simulink model "MCP_phase2_nonlinear_simulink"  (R2020a)
settings: Solver=VariableStepAuto  StartTime=0.0  StopTime=1000  RelTol=1e-3
values from neighbouring files (symbols this model uses):
  eq_values = zeros(4,1)    [MCP_phase2_nonlinear.m]
  h1_eq = 11.4    [MCP_phase2_linear.m]    (also in MCP_phase2_nonlinear.m)
  h2_eq = 11.6    [MCP_phase2_linear.m]    (also in MCP_phase2_nonlinear.m)
  h3_eq = 5.3    [MCP_phase2_linear.m]    (also in MCP_phase2_nonlinear.m)
  h4_eq = 4    [MCP_phase2_linear.m]    (also in MCP_phase2_nonlinear.m)
settings Model: Creator=rafiee  LastModifiedBy=Lenovo
settings DataIOCC: ReturnWorkspaceOutputs=off
settings DebuggingCC: ArithmeticOperatorsInVariantConditions=warning
settings SFSimCC: SimUseLocalCustomCode=off  CustomCodeUndefinedFunction=UseInterfaceOnly
settings RTWCC: RTWUseLocalCustomCode=off
settings CodeAppCC: StateflowObjectComments=on

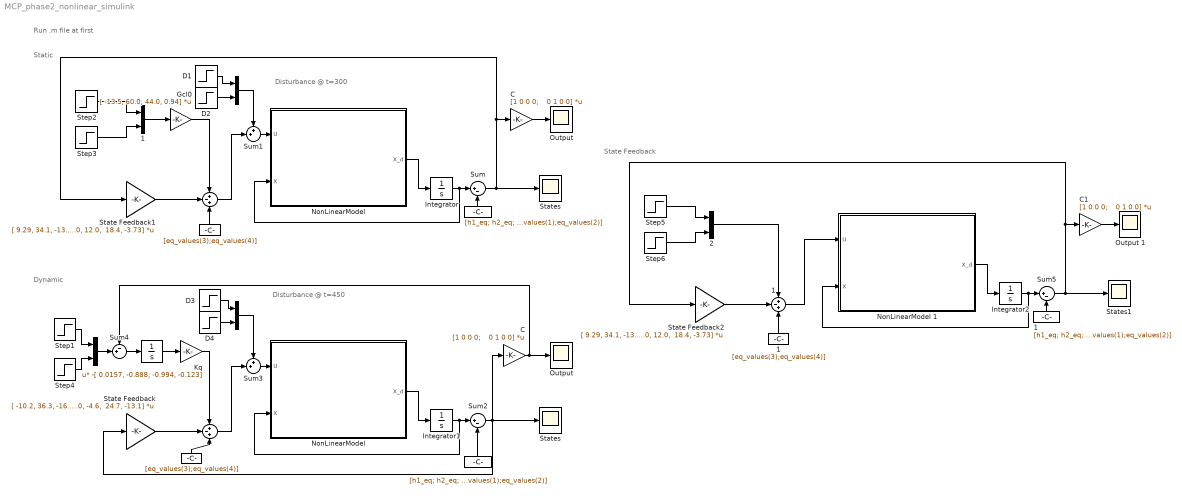
== system MCP_phase2_nonlinear_simulink ==
  note: State Feedback
  note: Run .m file at first
  note: Static
  note: Dynamic
  note: Disturbance @ t=450
  note: Disturbance @ t=300
  " " : Integrator
  " " : Sum  Inputs=+-+
  "      " : Concatenate
  "        " : Sum  Inputs=+-+
  "                        " : Constant  Value=[eq_values(3);eq_values(4)]
  "                             " : Constant  Value=[h1_eq; h2_eq; eq_values(1);eq_values(2)]
  " " : Constant  Value=[h1_eq; h2_eq; eq_values(1);eq_values(2)]
  "                                  " : Constant  Value=[eq_values(3);eq_values(4)]
  "                                                                   " : Concatenate
  "                                                                         " : Concatenate
  "                             1" : Constant  Value=[h1_eq; h2_eq; eq_values(1);eq_values(2)]
  "                        1" : Constant  Value=[eq_values(3);eq_values(4)]
  "        1" : Sum  Inputs=+-+
  "   1" : Concatenate
  "   2" : Concatenate
  C : Gain  Gain=|  Multiplication=Matrix(K*u)
      | [1 0 0 0;
      |    0 1 0 0]
  "C  " : Gain  Gain=|  Multiplication=Matrix(K*u)
      | [1 0 0 0;
      |    0 1 0 0]
  C1 : Gain  Gain=|  Multiplication=Matrix(K*u)
      | [1 0 0 0;
      |    0 1 0 0]
  D1 : Step  Time=300  After=4  SampleTime=0
  D2 : Step  Time=300  After=4  SampleTime=0
  D3 : Step  Time=450  After=4  SampleTime=0
  D4 : Step  Time=450  After=4  SampleTime=0
  Gcl0 : Gain  Gain=[ -13.5, 60.0; 44.0, 0.94]  Multiplication=Matrix(K*u)
  Integrator : Integrator  InitialCondition=[h1_eq;h2_eq;h3_eq;h4_eq]
  Integrator1 : Integrator  InitialCondition=[h1_eq;h2_eq;h3_eq;h4_eq]
  Integrator2 : Integrator  InitialCondition=[h1_eq;h2_eq;h3_eq;h4_eq]
  Kq : Gain  Gain=-[ 0.0157, -0.888; -0.994, -0.123]  Multiplication=Matrix(u*K)
  NonLinearModel : MATLAB Function  TreatAsAtomicUnit=on
  "NonLinearModel " : MATLAB Function  TreatAsAtomicUnit=on
  NonLinearModel 1 : MATLAB Function  TreatAsAtomicUnit=on
  "Output " : Scope
  Output 1 : Scope
  "Output  " : Scope
  "State Feedback " : Gain  Gain="[ -10.2, 36.3, -16.5,  24.5; 41.0, -4.6,  24.7, -13.1]"  Multiplication=Matrix(K*u)
  State Feedback1 : Gain  Gain="[ 9.29, 34.1, -13.6,  24.9; 23.0, 12.0,  18.4, -3.73]"  Multiplication=Matrix(K*u)
  State Feedback2 : Gain  Gain="[ 9.29, 34.1, -13.6,  24.9; 23.0, 12.0,  18.4, -3.73]"  Multiplication=Matrix(K*u)
  States : Scope
  "States " : Scope
  States1 : Scope
  Step{1..6} (6 alike) : Step  SampleTime=0
  Sum : Sum  Inputs=|+-
  Sum1 : Sum  Inputs=++|
  Sum2 : Sum  Inputs=|+-
  Sum3 : Sum  Inputs=++|
  Sum4 : Sum  Inputs=-+|
  Sum5 : Sum  Inputs=|+-
  wires:
  "                             "/1 -> Sum/2
  Integrator/1 -> Sum/1, "NonLinearModel "/2(X)
  Gcl0/1 -> "        "/1
  "NonLinearModel "/1(X_d) -> Integrator/1
  "   1"/1 -> Gcl0/1
  State Feedback1/1 -> "        "/2
  "                        "/1 -> "        "/3
  Step3/1 -> "   1"/2
  Step2/1 -> "   1"/1
  C/1 -> "Output "/1
  Sum/1 -> C/1, State Feedback1/1, States/1
  D1/1 -> "                                                                   "/1
  D2/1 -> "                                                                   "/2
  "                                                                   "/1 -> Sum1/1
  Sum1/1 -> "NonLinearModel "/1(U)
  "        "/1 -> Sum1/2
  "C  "/1 -> "Output  "/1, Sum4/1
  "      "/1 -> Sum4/2
  Sum4/1 -> " "/1
  Sum2/1 -> "State Feedback "/1, "States "/1, "C  "/1
  Step1/1 -> "      "/1
  Step4/1 -> "      "/2
  D3/1 -> "                                                                         "/1
  D4/1 -> "                                                                         "/2
  "State Feedback "/1 -> " "/2
  "                                                                         "/1 -> Sum3/1
  " "/1 -> Sum3/2
  NonLinearModel/1(X_d) -> Integrator1/1
  Kq/1 -> " "/1
  " "/1 -> Sum2/2
  " "/1 -> Kq/1
  Integrator1/1 -> Sum2/1, NonLinearModel/2(X)
  Sum3/1 -> NonLinearModel/1(U)
  "                                  "/1 -> " "/3
  Step6/1 -> "   2"/2
  Step5/1 -> "   2"/1
  C1/1 -> Output 1/1
  State Feedback2/1 -> "        1"/2
  Sum5/1 -> C1/1, State Feedback2/1, States1/1
  NonLinearModel 1/1(X_d) -> Integrator2/1
  Integrator2/1 -> Sum5/1, NonLinearModel 1/2(X)
  "                             1"/1 -> Sum5/2
  "                        1"/1 -> "        1"/3
  "   2"/1 -> "        1"/1
  "        1"/1 -> NonLinearModel 1/1(U)

== matlab function MCP_phase2_nonlinear_simulink/NonLinearModel ==
  data: U input; X input; X_d output
function X_d = non_linear_plant(U,X)
Area = [730 730 730 730]; % area of the tanks in cm^2
a = [2.10 2.14 2.2 2.3];  % area of the drain in cm^2
y = [0.3 0.35];           % y(1) = Ratio of flow in tank1 to flow in tank4                          % y(2) = Ratio of flow in tank2 to flow in tank3                   
k = [7.45 7.30];          % pump proportionality constants in cm^2/s
g = 981;                  % gravitational acceleration in cm/s^2

h1 = X(1);
h2 = X(2);
h3 = X(3);
h4 = X(4);
v1 = U(1);
v2 = U(2);

h1_d = -a(1)/Area(1)*sqrt(2*g*h1)+a(3)/Area(1)*sqrt(2*g*h3)+y(1)*k(1)/Area(1)*v1+0.00137;
h2_d = -a(2)/Area(2)*sqrt(2*g*h2)+a(4)/Area(2)*sqrt(2*g*h4)+y(2)*k(2)/Area(2)*v2+0.00137;
h3_d = -a(3)/Area(3)*sqrt(2*g*h3)+(1 - y(2))*k(2)/Area(3)*v2;
h4_d = -a(4)/Area(4)*sqrt(2*g*h4)+(1 - y(1))*k(1)/Area(4)*v1; 

X_d = [h1_d;h2_d;h3_d;h4_d];

== matlab function MCP_phase2_nonlinear_simulink/NonLinearModel 1 ==
  data: U input; X input; X_d output
function X_d   = non_linear_plant(U,X)
Area = [730 730 730 730]; % area of the tanks in cm^2
a = [2.10 2.14 2.2 2.3];  % area of the drain in cm^2
y = [0.3 0.35];           % y(1) = Ratio of flow in tank1 to flow in tank4
                          % y(2) = Ratio of flow in tank2 to flow in tank3                   
k = [7.45 7.30];          % pump proportionality constants in cm^2/s
g = 981;                  % gravitational acceleration in cm/s^2

h1 = X(1);
h2 = X(2);
h3 = X(3);
h4 = X(4);

v1 = U(1);
v2 = U(2);

h1_d = -a(1)/Area(1)*sqrt(2*g*h1)+a(3)/Area(1)*sqrt(2*g*h3)+y(1)*k(1)/Area(1)*v1+0.00137;
h2_d = -a(2)/Area(2)*sqrt(2*g*h2)+a(4)/Area(2)*sqrt(2*g*h4)+y(2)*k(2)/Area(2)*v2+0.00137;
h3_d = -a(3)/Area(3)*sqrt(2*g*h3)+(1 - y(2))*k(2)/Area(3)*v2;
h4_d = -a(4)/Area(4)*sqrt(2*g*h4)+(1 - y(1))*k(1)/Area(4)*v1;

X_d = [h1_d;h2_d;h3_d;h4_d];

== matlab function MCP_phase2_nonlinear_simulink/NonLinearModel  ==
  data: U input; X input; X_d output
function X_d   = non_linear_plant(U,X)
Area = [730 730 730 730]; % area of the tanks in cm^2
a = [2.10 2.14 2.2 2.3];  % area of the drain in cm^2
y = [0.3 0.35];           % y(1) = Ratio of flow in tank1 to flow in tank4                          % y(2) = Ratio of flow in tank2 to flow in tank3                   
k = [7.45 7.30];          % pump proportionality constants in cm^2/s
g = 981;                  % gravitational acceleration in cm/s^2

h1 = X(1);
h2 = X(2);
h3 = X(3);
h4 = X(4);

v1 = U(1);
v2 = U(2);

h1_d = -a(1)/Area(1)*sqrt(2*g*h1)+a(3)/Area(1)*sqrt(2*g*h3)+y(1)*k(1)/Area(1)*v1+0.00137;
h2_d = -a(2)/Area(2)*sqrt(2*g*h2)+a(4)/Area(2)*sqrt(2*g*h4)+y(2)*k(2)/Area(2)*v2+0.00137;
h3_d = -a(3)/Area(3)*sqrt(2*g*h3)+(1 - y(2))*k(2)/Area(3)*v2;
h4_d = -a(4)/Area(4)*sqrt(2*g*h4)+(1 - y(1))*k(1)/Area(4)*v1;

X_d = [h1_d;h2_d;h3_d;h4_d];
